simulink model "verify_Pressure_Drop_Fix_mdl"  (R2016b)
settings: Solver=VariableStepDiscrete  StartTime=0.0  StopTime=100  MaxStep=10  RelTol=1e-3  EnableMultiTasking=on
libraries: carnot x2, simulink x1
settings Model: Creator=drhf  LastModifiedBy=drhf
settings DataIOCC: LimitDataPoints=on  SaveFormat=Array  SignalLoggingSaveFormat=ModelDataLogs
settings OptimizationCC: ExpressionDepthLimit=2147483647  LifeSpan=inf
settings DebuggingCC: UnderspecifiedInitializationDetection=Classic  MergeDetectMultiDrivingBlocksExec=none  SolverPrmCheckMsg=warning  FcnCallInpInsideContextMsg=warning  StateNameClashWarn=warning  SFUnexpectedBacktrackingDiag=warning  SFNoUnconditionalDefaultTransitionDiag=warning  SFExecutionAtInitializationDiag=none
settings HardwareCC: ProdBitPerPointer=32  ProdBitPerSizeT=32  ProdBitPerPtrDiffT=32  ProdLargestAtomicFloat=None  ProdIntDivRoundTo=Undefined  ProdEndianess=Unspecified  ProdWordSize=32  ProdHWDeviceType=32-bit Generic
settings ModelReferenceCC: PropagateSignalLabelsOutOfModel=off
settings GRTTargetCC: TargetLangStandard=C89/C90 (ANSI)  GeneratePreprocessorConditionals=Disable all  CombineOutputUpdateFcns=off  GRTInterface=on
settings ConfigComp: CovMetricSettings=dw  CovHtmlReporting=on  CovSaveCumulativeToWorkspaceVar=on  CovSaveSingleToWorkspaceVar=on  CovExternalEMLEnable=off

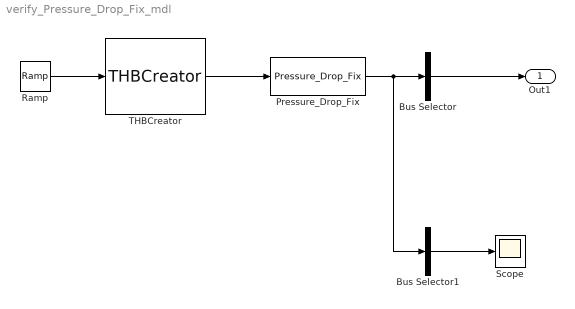
== system verify_Pressure_Drop_Fix_mdl ==
  Bus Selector : BusSelector  OutputSignals=MassFlow,Pressure,DPConstant,DPLinear,DPQuadratic  OutputAsBus=on
  Bus Selector1 : BusSelector  OutputSignals=Pressure  OutputAsBus=on
  Pressure_Drop_Fix : carnot/Basic/Pressure_Drop/Pressure_Drop_Fix  con=101  lin=202  qua=303
  Ramp : simulink/Sources/Ramp  slope=0.01  start=0  X0=0
  Scope : Scope
  THBCreator : carnot/Basic/Hydraulics/THBCreator  Inport_ID=off  Inport_T=off  Inport_mdot=on  Inport_p=off  Inport_type=off  Inport_mix=off  Inport_mix2=off  Inport_mix3=off  Inport_d=off  Inport_c=off  Inport_l=off  Inport_q=off  Inport_LH=off  Inport_H=off  ID=20001  T=20  mdot=0  p=1e5  FluidType=1  FluidMix=0  FluidMix2=0  FluidMix3=0  d=0.02  c=1  l=2  q=3  LH=0  H=0  Annotation_ID=off  Annotation_T=off  Annotation_mdot=off  Annotation_p=off  Annotation_type=off  Annotation_mix=off  Annotation_mix2=off  Annotation_mix3=off  Annotation_d=off  Annotation_c=off  Annotation_l=off  Annotation_q=off  Annotation_LH=off  Annotation_H=off
  Out1 : Outport
  wires:
  THBCreator/1 -> Pressure_Drop_Fix/1
  Pressure_Drop_Fix/1 -> Bus Selector1/1, Bus Selector/1
  Bus Selector/1 -> Out1/1
  Ramp/1 -> THBCreator/1
  Bus Selector1/1 -> Scope/1
